simulink model "fuzzy_controller_simulink"  (R2020a)
settings: Solver=ode23tb  StartTime=0.0  StopTime=100  RelTol=1e-3  EnableMultiTasking=on
libraries: fuzblock x1
settings Model: Creator=paulo.costa  LastModifiedBy=paulo
settings DataIOCC: LimitDataPoints=on  SaveFormat=Array  ReturnWorkspaceOutputs=off
settings OptimizationCC: LifeSpan=inf
settings DebuggingCC: UnderspecifiedInitializationDetection=Classic  MergeDetectMultiDrivingBlocksExec=none  SolverPrmCheckMsg=warning  StateNameClashWarn=warning  SFUnexpectedBacktrackingDiag=warning  SFNoUnconditionalDefaultTransitionDiag=warning  SFExecutionAtInitializationDiag=none  ArithmeticOperatorsInVariantConditions=warning
settings HardwareCC: ProdBitPerPointer=32  ProdBitPerSizeT=32  ProdBitPerPtrDiffT=32  ProdLargestAtomicFloat=None  ProdIntDivRoundTo=Undefined  ProdEndianess=Unspecified  ProdWordSize=32  ProdHWDeviceType=32-bit Generic
settings ModelReferenceCC: PropagateSignalLabelsOutOfModel=off
settings SFSimCC: SimUseLocalCustomCode=off  CustomCodeUndefinedFunction=UseInterfaceOnly
settings RTWCC: RTWUseLocalCustomCode=off
settings CodeAppCC: StateflowObjectComments=on
settings GRTTargetCC: TargetLangStandard=C89/C90 (ANSI)
settings ConfigComp: CovMetricSettings=dw  CovHtmlReporting=on  CovSaveCumulativeToWorkspaceVar=on  CovSaveSingleToWorkspaceVar=on  CovExternalEMLEnable=off

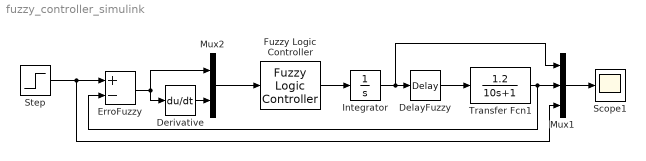
== system fuzzy_controller_simulink ==
  DelayFuzzy : TransportDelay  DelayTime=2
  Derivative : Derivative
  ErroFuzzy : Sum  Inputs=+-
  Fuzzy Logic Controller : fuzblock/Fuzzy Logic  Controller  FIS=fuzzy_controller  OutputSampleNumber=101  DataType=double  FuzzifiedInputs=off  RuleFiringStrengths=off  RuleOutputs=off  AggregatedOutputs=off  SimulateUsing=Interpreted execution  OutOfRangeInputValueMessage=warning  NoRuleFiredMessage=warning  EmptyOutputFuzzySetMessage=warning
  Integrator : Integrator
  Mux1 : Mux  Inputs=3
  Mux2 : Mux  Inputs=2
  Scope1 : Scope
  Step : Step  SampleTime=0
  Transfer Fcn1 : TransferFcn  Numerator=[1.2]  Denominator=[10 1]
  wires:
  Mux1/1 -> Scope1/1
  Step/1 -> Mux1/3, ErroFuzzy/1
  Fuzzy Logic Controller/1 -> Integrator/1
  Derivative/1 -> Mux2/2
  ErroFuzzy/1 -> Mux2/1, Derivative/1
  Mux2/1 -> Fuzzy Logic Controller/1
  Integrator/1 -> Mux1/1, DelayFuzzy/1
  DelayFuzzy/1 -> Transfer Fcn1/1
  Transfer Fcn1/1 -> Mux1/2, ErroFuzzy/2
